simulink model "P3Simulink"  (R2025a)
settings: Solver=VariableStepAuto  StartTime=0.0  StopTime=10  RelTol=1e-3
InitFcn:
  | m1=290;
  | b1=1000;
  | m2=59;
  | k1=16182;
  | f=0;
  | k2=19000;
  | z1 =0.05;
  | z2 =0;
settings Model: Creator=sanch  LastModifiedBy=ismae

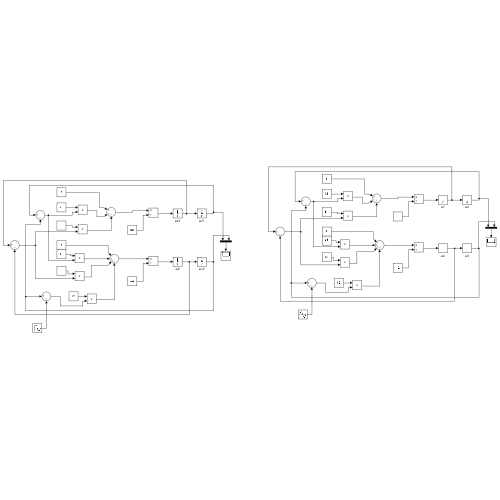
[thumbnail: Simulink's stored preview of the top-level diagram]
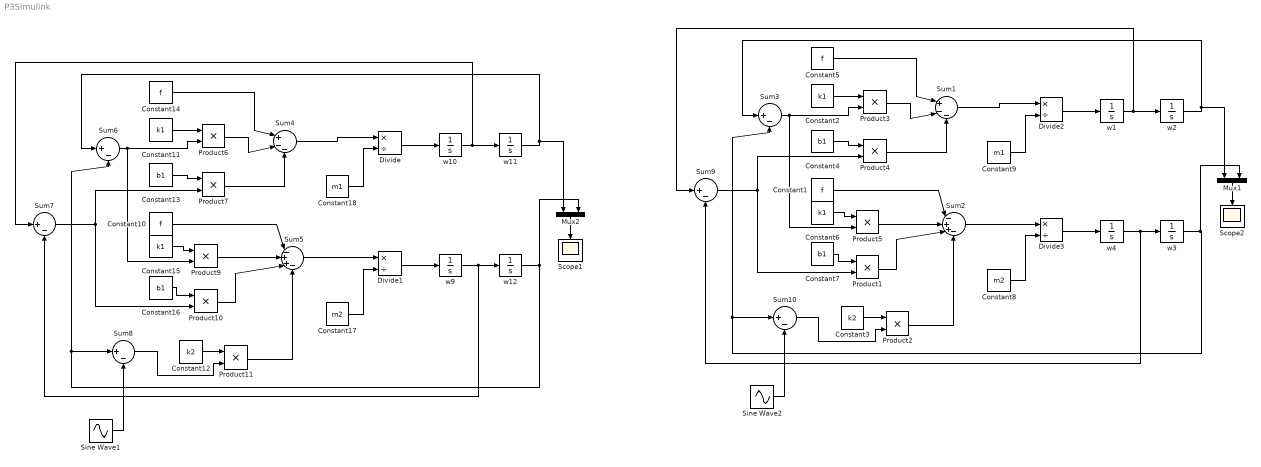
== system P3Simulink ==
  Constant{1,5,10,14} (4 alike) : Constant  Value=f
  Constant{2,6,11,15} (4 alike) : Constant  Value=k1
  Constant12 : Constant  Value=k2
  Constant{4,7,13,16} (4 alike) : Constant  Value=b1
  Constant17 : Constant  Value=m2
  Constant18 : Constant  Value=m1
  Constant3 : Constant  Value=k2
  Constant8 : Constant  Value=m2
  Constant9 : Constant  Value=m1
  Divide{,1..3} (4 alike) : Product  Inputs=*/
  Mux1 : Mux  Inputs=2
  Mux2 : Mux  Inputs=2
  Product{1..7,9..11} (10 alike) : Product
  Scope1 : Scope
      settings: ActiveDisplayYMinimum=-0.24199643125966608  ActiveDisplayYMaximum=0.2944675380596582
  Scope2 : Scope
      settings: ActiveDisplayYMinimum=-0.012359577489778284  ActiveDisplayYMaximum=0.0218471149345304
  Sine Wave1 : Sin  Amplitude=0.05  Frequency=0.5*pi  SampleTime=0
  Sine Wave2 : Sin  Amplitude=0.05  Frequency=20*pi  SampleTime=0
  Sum1 : Sum  Inputs=|+--
  Sum{3,6..10} (6 alike) : Sum  Inputs=|+-
  Sum2 : Sum  Inputs=|-++-
  Sum4 : Sum  Inputs=|+--
  Sum5 : Sum  Inputs=|-++-
  w{1..4,9..12} (8 alike) : Integrator
  wires:
  Constant11/1 -> Product6/1
  Constant14/1 -> Sum4/1
  Product6/1 -> Sum4/2
  Constant13/1 -> Product7/1
  Product7/1 -> Sum4/3
  Constant10/1 -> Sum5/1
  Constant15/1 -> Product9/1
  Product9/1 -> Sum5/2
  Constant16/1 -> Product10/1
  Product10/1 -> Sum5/3
  Product11/1 -> Sum5/4
  Constant17/1 -> Divide1/2
  Sum5/1 -> Divide1/1
  Constant18/1 -> Divide/2
  Divide1/1 -> w9/1
  w10/1 -> Sum7/1, w11/1
  w9/1 -> w12/1, Sum7/2
  Sum6/1 -> Product9/2, Product6/2
  Sum7/1 -> Product10/2, Product7/2
  Constant12/1 -> Product11/1
  Sine Wave1/1 -> Sum8/2
  w12/1 -> Mux2/2, Sum8/1, Sum6/2
  w11/1 -> Mux2/1, Sum6/1
  Sum4/1 -> Divide/1
  Divide/1 -> w10/1
  Sum8/1 -> Product11/2
  Mux2/1 -> Scope1/1
  Mux1/1 -> Scope2/1
  Sum10/1 -> Product2/2
  Divide2/1 -> w1/1
  Sum1/1 -> Divide2/1
  w2/1 -> Sum3/1, Mux1/1
  w3/1 -> Sum3/2, Sum10/1, Mux1/2
  Sine Wave2/1 -> Sum10/2
  Constant3/1 -> Product2/1
  Sum9/1 -> Product4/2, Product1/2
  Sum3/1 -> Product3/2, Product5/2
  w4/1 -> Sum9/2, w3/1
  w1/1 -> w2/1, Sum9/1
  Divide3/1 -> w4/1
  Constant9/1 -> Divide2/2
  Sum2/1 -> Divide3/1
  Constant8/1 -> Divide3/2
  Product2/1 -> Sum2/4
  Product1/1 -> Sum2/3
  Constant7/1 -> Product1/1
  Product5/1 -> Sum2/2
  Constant6/1 -> Product5/1
  Constant1/1 -> Sum2/1
  Product4/1 -> Sum1/3
  Constant4/1 -> Product4/1
  Product3/1 -> Sum1/2
  Constant5/1 -> Sum1/1
  Constant2/1 -> Product3/1
